simulink model "Multirate"  (R2014a)
settings: Solver=ode1  StartTime=0.0  StopTime=10.0  FixedStep=0.01  RelTol=1e-3
libraries: mbed_lib x3
settings Model: Creator=BassAllUser  LastModifiedBy=BassUser
settings OptimizationCC: OptimizeModelRefInitCode=on  LifeSpan=1
settings HardwareCC: ProdBitPerInt=16  ProdBitPerPointer=8  ProdIntDivRoundTo=Zero  ProdEndianess=LittleEndian  ProdWordSize=8  ProdHWDeviceType=Atmel->AVR
settings RTWCC: SystemTargetFile=mbed.tlc  GenCodeOnly=on  PackageGeneratedCodeAndArtifacts=on  PackageName=SimulinkExportPackage  TemplateMakefile=mbed.tmf  Description=mbed  GenerateReport=on  ProcessScript=mbed_make_rtw_hook  IncludeHyperlinkInReport=on  LaunchReport=on  TargetLang=C++
settings CodeAppCC: IgnoreCustomStorageClasses=off
settings STFCustomTargetCC: TargetLibSuffix=.a  GenerateSampleERTMain=on  ConcurrentExecutionCompliant=off  GeneratePreprocessorConditionals=Use local settings  CombineOutputUpdateFcns=on  ERTCustomFileBanners=on  SupportNonInlinedSFcns=off  MATLABClassNameForMDSCustomization=Simulink.SoftwareTarget.ERTCustomization  GRTInterface=off  SystemTargetFile=mbed.tlc
settings GRTTargetCC: TargetLibSuffix=.a  GenerateSampleERTMain=on  ParMdlRefBuildCompliant=off  CompOptLevelCompliant=off  ConcurrentExecutionCompliant=off  GeneratePreprocessorConditionals=Use local settings  ERTCustomFileBanners=on  MatFileLogging=off  SupportNonInlinedSFcns=off  MATLABClassNameForMDSCustomization=Simulink.SoftwareTarget.ERTCustomization  CPPClassGenCompliant=off

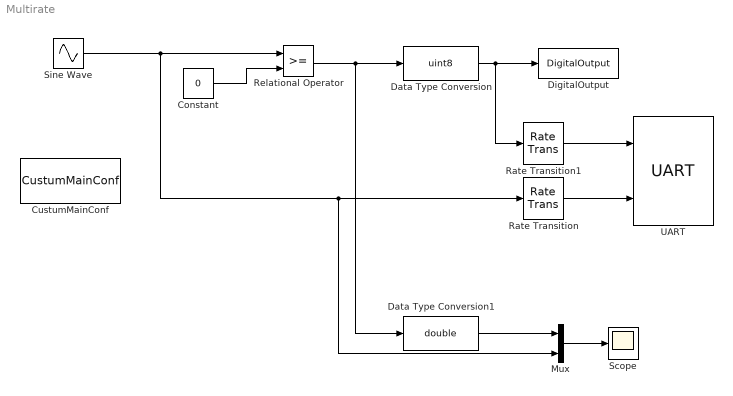
== system Multirate ==
  Constant : Constant  Value=0
  CustumMainConf : mbed_lib/CustumMainConf  P1=main.c  P2=0
  Data Type Conversion : DataTypeConversion  OutDataTypeStr=uint8
  Data Type Conversion1 : DataTypeConversion  OutDataTypeStr=double
  DigitalOutput : mbed_lib/DigitalOutput  SParameter1='LED1'  SParameter2=-1
  Mux : Mux  Inputs=2
  Rate Transition : RateTransition
  Rate Transition1 : RateTransition
  Relational Operator : RelationalOperator  OutDataTypeStr=boolean
  Scope : Scope
  Sine Wave : Sin  SampleTime=0
  UART : mbed_lib/UART  SFunctionSpec=double y1 = dummy(int8 p1,int8 p2,int8 p3)  SParameter1=2  SParameter2=led -> %d ; sin -> %4.2f\n  SParameter3=1
  wires:
  Data Type Conversion/1 -> Rate Transition1/1, DigitalOutput/1
  Constant/1 -> Relational Operator/2
  Sine Wave/1 -> Mux/2, Rate Transition/1, Relational Operator/1
  Rate Transition/1 -> UART/2
  Mux/1 -> Scope/1
  Rate Transition1/1 -> UART/1
  Relational Operator/1 -> Data Type Conversion1/1, Data Type Conversion/1
  Data Type Conversion1/1 -> Mux/1
